simulink model "sim_DC_Motor_FOM_verification"  (R2024b)
settings: Solver=VariableStepAuto  StartTime=0.0  StopTime=Tsim  RelTol=1e-3
values from neighbouring files (symbols this model uses):
  A_verif = A_hat    [main_SysId_DC_Motor_LS_Full_model.m]    (also in main_SysId_DC_Motor_LS_KF_RO_model.m; main_SysId_DC_Motor_LS_RO_model.m; main_SysId_DC_Motor_RLS_RO_model.m)
  B_verif = B_hat    [main_SysId_DC_Motor_LS_Full_model.m]    (also in main_SysId_DC_Motor_LS_KF_RO_model.m; main_SysId_DC_Motor_LS_RO_model.m; main_SysId_DC_Motor_RLS_RO_model.m)
  ts = 1/fs    (= 0.01)    [main_SysId_DC_Motor_LS_Full_model.m]    (also in main_SysId_DC_Motor_LS_KF_RO_model.m = 0.005; main_SysId_DC_Motor_LS_RO_model.m = 0.005; main_SysId_DC_Motor_RLS_RO_model.m = 0.005)
  Vpeak = 2    [main_SysId_DC_Motor_LS_Full_model.m]    (also in main_SysId_DC_Motor_LS_KF_RO_model.m = 5; main_SysId_DC_Motor_LS_RO_model.m = 3; main_SysId_DC_Motor_RLS_RO_model.m = 3)
settings Model: Creator=ricardoaguilera  LastModifiedBy=ricardoaguilera
settings SolverCC: AutoInsertRateTranBlk=on
settings DataIOCC: ReturnWorkspaceOutputs=off

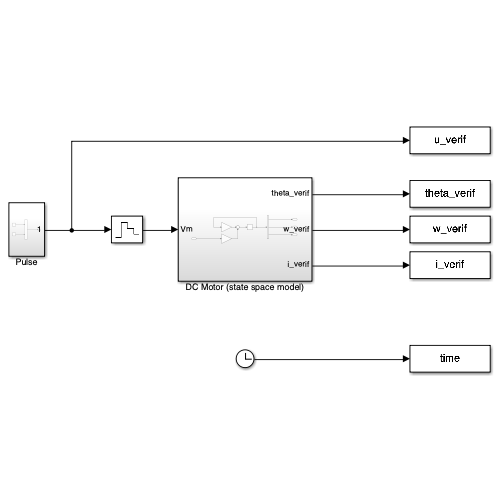
[thumbnail: Simulink's stored preview of the top-level diagram]
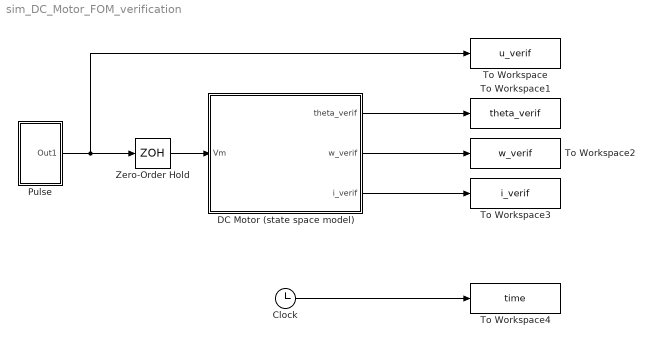
== system sim_DC_Motor_FOM_verification ==
  Clock : Clock
  DC Motor (state space model) : Subsystem
  Pulse : Subsystem
  To Workspace : ToWorkspace  VariableName=u_verif  SampleTime=ts
  To Workspace1 : ToWorkspace  VariableName=theta_verif  SampleTime=ts
  To Workspace2 : ToWorkspace  VariableName=w_verif  SampleTime=ts
  To Workspace3 : ToWorkspace  VariableName=i_verif  SampleTime=ts
  To Workspace4 : ToWorkspace  VariableName=time  SampleTime=ts
  Zero-Order Hold : ZeroOrderHold  SampleTime=ts
  wires:
  Pulse/1(Out1) -> Zero-Order Hold/1, To Workspace/1
  DC Motor (state space model)/1(theta_verif) -> To Workspace1/1
  DC Motor (state space model)/2(w_verif) -> To Workspace2/1
  Clock/1 -> To Workspace4/1
  Zero-Order Hold/1 -> DC Motor (state space model)/1(Vm)
  DC Motor (state space model)/3(i_verif) -> To Workspace3/1

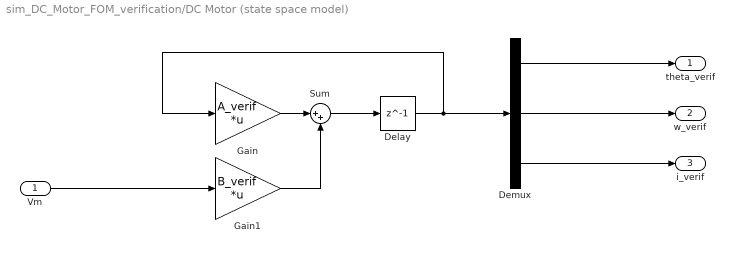
== system sim_DC_Motor_FOM_verification/DC Motor (state space model) ==
  Vm : Inport
  Delay : Delay  DelayLength=1
  Demux : Demux  Outputs=3
  Gain : Gain  Gain=A_verif  Multiplication=Matrix(K*u)
  Gain1 : Gain  Gain=B_verif  Multiplication=Matrix(K*u)
  Sum : Sum  Inputs=|++
  theta_verif : Outport
  w_verif : Outport  Port=2
  i_verif : Outport  Port=3
  wires:
  Delay/1 -> Gain/1, Demux/1
  Sum/1 -> Delay/1
  Vm/1 -> Gain1/1
  Gain1/1 -> Sum/2
  Gain/1 -> Sum/1
  Demux/1 -> theta_verif/1
  Demux/2 -> w_verif/1
  Demux/3 -> i_verif/1

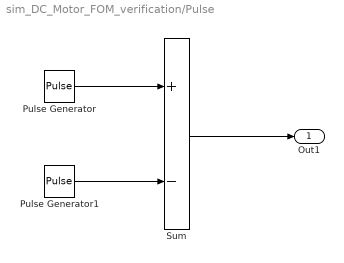
== system sim_DC_Motor_FOM_verification/Pulse ==
  Pulse Generator : DiscretePulseGenerator  PulseType=Time based  Amplitude=Vpeak  Period=10  PulseWidth=10  PhaseDelay=2
  Pulse Generator1 : DiscretePulseGenerator  PulseType=Time based  Amplitude=Vpeak  Period=10  PulseWidth=10  PhaseDelay=6
  Sum : Sum  Inputs=+-
  Out1 : Outport
  wires:
  Sum/1 -> Out1/1
  Pulse Generator/1 -> Sum/1
  Pulse Generator1/1 -> Sum/2
